simulink model "multi_level_new"  (R2020a)
settings: Solver=VariableStepAuto  StartTime=0.0  StopTime=0.1  RelTol=1e-3
undefined symbols (not defined in the file): V
libraries: powerlib x19
settings Model: Creator=hp  LastModifiedBy=hp

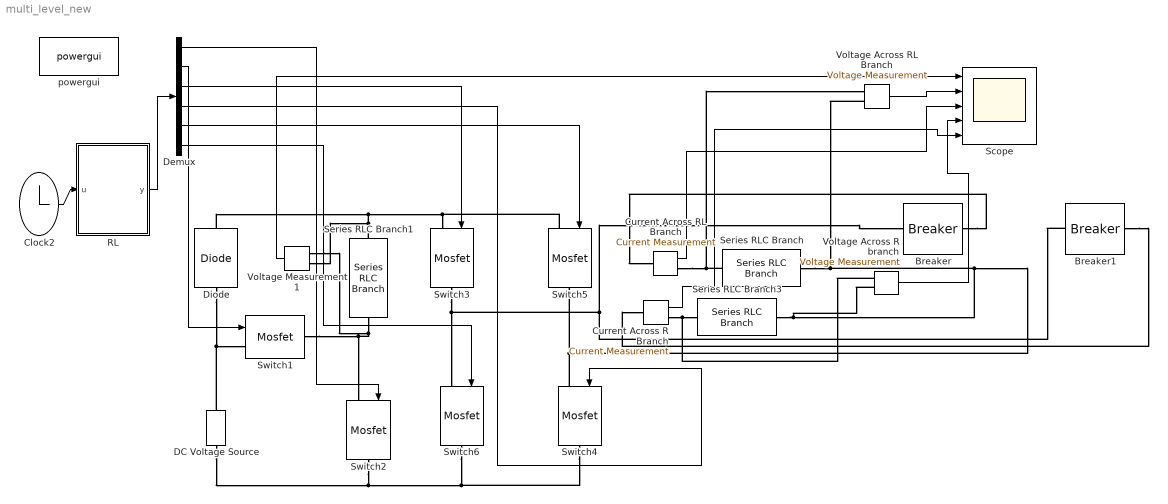
== system multi_level_new ==
  Breaker : powerlib/Elements/Breaker  InitialState=0  SwitchingTimes=[0.04 1]  External=off  BreakerResistance=0.01  SnubberResistance=1e6  SnubberCapacitance=inf  Measurements=None  MoreParameters=on  NoBreakLoop=off
  Breaker1 : powerlib/Elements/Breaker  InitialState=0  SwitchingTimes=[0 0.04]  External=off  BreakerResistance=0.01  SnubberResistance=1e6  SnubberCapacitance=inf  Measurements=None  MoreParameters=on  NoBreakLoop=off
  Clock2 : Clock
  Current Across R Branch : powerlib/Measurements/Current Measurement  PhasorSimulation=off  OutputType=Complex  PSBequivalent=0
  Current Across RL Branch : powerlib/Measurements/Current Measurement  PhasorSimulation=off  OutputType=Complex  PSBequivalent=0
  DC Voltage Source : powerlib/Electrical Sources/DC Voltage Source  Amplitude=V  Measurements=None
  Demux : Demux  Outputs=6
  Diode : powerlib/Power Electronics/Diode  Ron=0.001  Lon=0  Vf=0.8  IC=0  UseSnubber=0  Rs=500  Cs=250e-9  Measurements=off
  RL : MATLAB Function  TreatAsAtomicUnit=on
  Scope : Scope  NumInputPorts=5
  Series RLC Branch : powerlib/Elements/Series RLC Branch  LConnTagsString=__new0  RConnTagsString=__new0  BranchType=RL  Resistance=100  Inductance=0.5  SetiL0=off  InitialCurrent=0  Capacitance=1e-6  Setx0=off  InitialVoltage=0  Measurements=None
  Series RLC Branch1 : powerlib/Elements/Series RLC Branch  LConnTagsString=__new0  RConnTagsString=__new0  BranchType=C  Resistance=1  Inductance=1e-3  SetiL0=off  InitialCurrent=0  Capacitance=2200e-6  Setx0=on  InitialVoltage=0  Measurements=None
  Series RLC Branch3 : powerlib/Elements/Series RLC Branch  LConnTagsString=__new0  RConnTagsString=__new0  BranchType=R  Resistance=100  Inductance=0.5  SetiL0=off  InitialCurrent=0  Capacitance=1e-6  Setx0=off  InitialVoltage=0  Measurements=None
  Switch{1..6} (6 alike) : powerlib/Power Electronics/Mosfet  Ron=0.1  Lon=0  Rd=0.01  Vfd=0  IC=0  Rs=1e5  Cs=inf  Measurements=off
  Voltage Across R branch : powerlib/Measurements/Voltage Measurement  PhasorSimulation=off  OutputType=Complex  PSBequivalent=0
  Voltage Across RL Branch : powerlib/Measurements/Voltage Measurement  PhasorSimulation=off  OutputType=Complex  PSBequivalent=0
  Voltage Measurement1 : powerlib/Measurements/Voltage Measurement  PhasorSimulation=off  OutputType=Complex  PSBequivalent=0
  powergui : powerlib/powergui  Priority=1  SimulationMode=Discrete  SampleTime=50e-6  frequency=60  Iterations=50  frequencyindice=0  Pbase=100e6  ErrMax=1e-4  UnitsV=kV  UnitsW=MW  buscounter=0  FunctionMessages=off  echomessages=off  EnableUseOfTLC=off  CurrentSourceSwitches=off  DisableSnubberDevices=off  DisableRonSwitches=off  DisableVfSwitches=off  DisplayEquations=off  AutomaticDiscreteSolvers=off  SolverType=Tustin/Backward Euler (TBE)  Interpol=off  ExternalGateDelay=off  methode=off  Ts=100  x0status=blocks  SPID=on  SwTol=0  HookPort=off  NonlinearTolerance=1e-4  nMaxIteration=100  ContinueOnMaxIteration=off  RestoreLinks=warning  ResistiveCurrentMeasurement=off  Frange=[0:2:500]  Ylog=off  Xlog=on  ShowGrid=off  save=off  variable=ZData  structure=0  ZoomFFT=off  StartTime=0.0  cycles=1  DisplayStyle=1  fundamental=60  FreqAxis=off  MaxFrequency=1000  frequencyindicesteady=1  RmsSteady=1  display=off
  wires:
  Demux/2 -> Switch1/1
  Demux/1 -> Switch2/1
  Demux/6 -> Switch6/1
  Voltage Measurement1/1 -> Scope/1
  Demux/4 -> Switch4/1
  Voltage Across RL Branch/1 -> Scope/2
  Current Across RL Branch/1 -> Scope/3
  Clock2/1 -> RL/1(u)
  RL/1(y) -> Demux/1
  Demux/3 -> Switch3/1
  Demux/5 -> Switch5/1
  Current Across R Branch/1 -> Scope/5
  Voltage Across R branch/1 -> Scope/4
  connections:
  Switch5/LConn1 -- Voltage Measurement1/LConn1 -- Series RLC Branch1/LConn1 -- Diode/RConn1 -- Switch3/LConn1
  Switch3/RConn1 -- Breaker/LConn1 -- Breaker1/LConn1 -- Switch6/LConn1
  Switch6/RConn1 -- Switch2/RConn1 -- DC Voltage Source/LConn1 -- Switch4/RConn1
  Switch4/LConn1 -- Switch5/RConn1 -- Voltage Across R branch/LConn2 -- Series RLC Branch3/RConn1 -- Series RLC Branch/RConn1 -- Voltage Across RL Branch/LConn2
  Diode/LConn1 -- DC Voltage Source/RConn1 -- Switch1/LConn1
  Switch1/RConn1 -- Voltage Measurement1/LConn2 -- Series RLC Branch1/RConn1 -- Switch2/LConn1
  Series RLC Branch/LConn1 -- Current Across RL Branch/RConn1 -- Voltage Across RL Branch/LConn1
  Current Across R Branch/RConn1 -- Voltage Across R branch/LConn1 -- Series RLC Branch3/LConn1
  Breaker/RConn1 -- Current Across RL Branch/LConn1
  Breaker1/RConn1 -- Current Across R Branch/LConn1

== matlab function multi_level_new/RL ==
  data: u input; y output
function y = fcn(u)
% #eml
a=mod(u,0.02);
b=abs(sin(2*pi*50*a));
d=sin(2*pi*50*a);
x=0.3;
if d>0
    c=1;
else
    c=0;
end

if b<x/2          % Level 0                                        
    s1=0;
    s2=0;
    T1=1;
    T2=0;
    T3=1;
    T4=0;
   
elseif b<(x+1)/2      % Level +1
    s1=1;
    s2=0;
    T1=1;
    T2=1;
    T3=0;
    T4=0;

   
elseif b<(x+2)/2      % Level +2
    s1=0;
    s2=1;
    T1=1;
    T2=1;
    T3=0;
    T4=0;
 
else              % Level 0
    s1=0;
    s2=0;
    T1=1;
    T2=0;
    T3=1;
    T4=0;
        
end

    
    if c==1
        
    y = [s1,s2,T1,T2,T3,T4];
    else
        
        
    % For negative levels
            
   if b<x/2          % Level 0
    s1=0;
    s2=0;
    T1=0;
    T2=1;
    T3=0;
    T4=1;


elseif b<(x+1)/2      % Level -1
    s1=1;
    s2=0;
    T1=0;
    T2=0;
    T3=1;
    T4=1;

elseif b<(x+2)/2      % Level -2
    s1=0;
    s2=1;
    T1=0;
    T2=0;
    T3=1;
    T4=1;

else              % Level 0
    s1=0;
    s2=0;
    T1=0;
    T2=1;
    T3=0;
    T4=1;
  
        
   end

    y = [s1,s2,T1,T2,T3,T4];
    end
